simulink model "Model_TranslationEngine64"  (R2022b)
settings: Solver=FixedStepDiscrete  StartTime=0.0  StopTime=5  RelTol=1e-3  EnableMultiTasking=on
InitFcn:
  | % Initialize model
  | ModelSettings=BTConfig.GetModelSettings();
  | 
  | ModelSettings.Validate();
  | 
  | ModelInit;
  | 
  | 
  | % load library data
  | GainLibrary_data;
  | % Load saved values from partition process
  | CapturedConstMask.LoadMapFromFile(bdroot)
StartFcn:
  | % make sure all the simulated RTC requests are found
  | %RTC_SIM_OBJ.ValidateREQs();
undefined symbols (not defined in the file or in its folder): AA, BPLP, Column, NumHFRefBPF, NumHFRefLPF, NumMusicChannels, Row, VolumeMuteConfig
libraries: TuneVar x925, TOP x490, FeaturePath x111, CapturedConstLib x52
(part 28 of 34)

== system Model_TranslationEngine64/ModelPreAmp/DecRate/Medusa5H1/MedusaHoligram/Medusa5H1 Part 3/On/Full-rate Mixer/Full-Rate Mixer with CAE & Fade Ramper/Fade Tuning/Forward Downmix Threshold ==
  TOP : TOP/TOP  TriggerInit=[440 20 585 80]  TopName=ForwardDownmixThreshold  DataTypeOut=single  BankNumber=0  PreOverlay=false  PostOverlay=false  Role=Automatic
      settings: SourceProductName=Bose Talaria
  TranslateTrigger : TuneVar/TranslateTrigger  TriggerInit=[291 -100 329 -45]
      settings: SourceProductName=Bose Talaria
  Trivial Translation : MATLAB Function  TreatAsAtomicUnit=on
  Tune Variable : TuneVar/TuneVar  TuneName=ForwardDownmixThreshold  SpecifyMaxSize=off  VariableDim=1 (Row)  MaxSize=[1 1]  TunabilityNumber=1  MinValue=[0]  MaxValue=[1]  TriggerInit=[-80 25 90 75]  MaskValue=MedusaFRMTune.ForwardDownmixThreshold
      settings: SourceProductName=Bose Talaria
  wires:
  Tune Variable/1 -> Trivial Translation/1(ForwardDownmixThreshold)  "ForwardDownmixThreshold"
  Trivial Translation/1(TOP) -> TOP/1
  TranslateTrigger/1 -> Trivial Translation/Trigger

== system Model_TranslationEngine64/ModelPreAmp/DecRate/Medusa5H1/MedusaHoligram/Medusa5H1 Part 3/On/Full-rate Mixer/Full-Rate Mixer with CAE & Fade Ramper/Fade Tuning/Foward Downmix Max ==
  TOP : TOP/TOP  TriggerInit=[440 20 585 80]  TopName=ForwardDownmixMax  DataTypeOut=single  BankNumber=0  PreOverlay=false  PostOverlay=false  Role=Automatic
      settings: SourceProductName=Bose Talaria
  TranslateTrigger : TuneVar/TranslateTrigger  TriggerInit=[286 -100 324 -45]
      settings: SourceProductName=Bose Talaria
  Trivial Translation : MATLAB Function  TreatAsAtomicUnit=on
  Tune Variable : TuneVar/TuneVar  TuneName=ForwardDownmixMax  SpecifyMaxSize=off  VariableDim=1 (Row)  MaxSize=[1 1]  TunabilityNumber=1  MinValue=[0]  MaxValue=[1]  TriggerInit=[-70 25 100 75]  MaskValue=MedusaFRMTune.ForwardDownmixMax
      settings: SourceProductName=Bose Talaria
  wires:
  Tune Variable/1 -> Trivial Translation/1(ForwardDownmixMax)  "ForwardDownmixMax"
  Trivial Translation/1(TOP) -> TOP/1
  TranslateTrigger/1 -> Trivial Translation/Trigger

== system Model_TranslationEngine64/ModelPreAmp/DecRate/Medusa5H1/MedusaHoligram/Medusa5H1 Part 3/On/Full-rate Mixer/Full-Rate Mixer with CAE & Fade Ramper/SLC Tuning/Detent Level CS ==
  TOP : TOP/TOP  TriggerInit=[440 -15 585 45]  TopName=DetentLevel_CS  DataTypeOut=single  BankNumber=0  PreOverlay=false  PostOverlay=false  Role=Automatic
      settings: SourceProductName=Bose Talaria
  TOP1 : TOP/TOP  TriggerInit=[440 55 585 115]  TopName=DetentLevel_CS_CAE  DataTypeOut=single  BankNumber=0  PreOverlay=false  PostOverlay=false  Role=Automatic
      settings: SourceProductName=Bose Talaria
  TranslateTrigger : TuneVar/TranslateTrigger  TriggerInit=[306 -100 344 -45]
      settings: SourceProductName=Bose Talaria
  Trivial Translation : MATLAB Function  TreatAsAtomicUnit=on
  Tune Variable : TuneVar/TuneVar  TuneName=DetentLevel_CS  SpecifyMaxSize=off  VariableDim=1 (Row)  MaxSize=[1 1]  TunabilityNumber=1  MinValue=[0]  MaxValue=[1]  TriggerInit=[-35 25 135 75]  MaskValue=MedusaFRMTune.detentGain_CS
      settings: SourceProductName=Bose Talaria
  wires:
  Trivial Translation/2(TOP_CAE) -> TOP1/1
  TranslateTrigger/1 -> Trivial Translation/Trigger
  Trivial Translation/1(TOP) -> TOP/1
  Tune Variable/1 -> Trivial Translation/1(detentGain_CS)  "DetentLevel_CS"

== system Model_TranslationEngine64/ModelPreAmp/DecRate/Medusa5H1/MedusaHoligram/Medusa5H1 Part 3/On/Full-rate Mixer/Full-Rate Mixer with CAE & Fade Ramper/SLC Tuning/Detent Level Left ==
  TOP : TOP/TOP  TriggerInit=[440 -15 585 45]  TopName=DetentLevel_Left  DataTypeOut=single  BankNumber=0  PreOverlay=false  PostOverlay=false  Role=Automatic
      settings: SourceProductName=Bose Talaria
  TOP1 : TOP/TOP  TriggerInit=[440 55 585 115]  TopName=DetentLevel_Left_CAE  DataTypeOut=single  BankNumber=0  PreOverlay=false  PostOverlay=false  Role=Automatic
      settings: SourceProductName=Bose Talaria
  TranslateTrigger : TuneVar/TranslateTrigger  TriggerInit=[306 -100 344 -45]
      settings: SourceProductName=Bose Talaria
  Trivial Translation : MATLAB Function  TreatAsAtomicUnit=on
  Tune Variable : TuneVar/TuneVar  TuneName=DetentLevel_Left  SpecifyMaxSize=off  VariableDim=1 (Row)  MaxSize=[1 1]  TunabilityNumber=1  MinValue=[0]  MaxValue=[1]  TriggerInit=[-65 25 105 75]  MaskValue=MedusaFRMTune.detentGain_Left
      settings: SourceProductName=Bose Talaria
  wires:
  Trivial Translation/2(TOP_CAE) -> TOP1/1
  TranslateTrigger/1 -> Trivial Translation/Trigger
  Trivial Translation/1(TOP) -> TOP/1
  Tune Variable/1 -> Trivial Translation/1(detentGain_Left)  "DetentLevel_Left"

== system Model_TranslationEngine64/ModelPreAmp/DecRate/Medusa5H1/MedusaHoligram/Medusa5H1 Part 3/On/Full-rate Mixer/Full-Rate Mixer with CAE & Fade Ramper/SLC Tuning/Detent Level Right ==
  TOP : TOP/TOP  TriggerInit=[440 -15 585 45]  TopName=DetentLevel_Right  DataTypeOut=single  BankNumber=0  PreOverlay=false  PostOverlay=false  Role=Automatic
      settings: SourceProductName=Bose Talaria
  TOP1 : TOP/TOP  TriggerInit=[440 55 585 115]  TopName=DetentLevel_Right_CAE  DataTypeOut=single  BankNumber=0  PreOverlay=false  PostOverlay=false  Role=Automatic
      settings: SourceProductName=Bose Talaria
  TranslateTrigger : TuneVar/TranslateTrigger  TriggerInit=[306 -100 344 -45]
      settings: SourceProductName=Bose Talaria
  Trivial Translation : MATLAB Function  TreatAsAtomicUnit=on
  Tune Variable : TuneVar/TuneVar  TuneName=DetentLevel_Right  SpecifyMaxSize=off  VariableDim=1 (Row)  MaxSize=[1 1]  TunabilityNumber=1  MinValue=[0]  MaxValue=[1]  TriggerInit=[-60 25 110 75]  MaskValue=MedusaFRMTune.detentGain_Right
      settings: SourceProductName=Bose Talaria
  wires:
  Trivial Translation/2(TOP_CAE) -> TOP1/1
  TranslateTrigger/1 -> Trivial Translation/Trigger
  Trivial Translation/1(TOP) -> TOP/1
  Tune Variable/1 -> Trivial Translation/1(detentGain_Right)  "DetentLevel_Right"

== system Model_TranslationEngine64/ModelPreAmp/DecRate/Medusa5H1/MedusaHoligram/Medusa5H1 Part 3/On/Full-rate Mixer/Full-Rate Mixer with CAE & Fade Ramper/SLC Tuning/Interpolation Method ==
  TOP : TOP/TOP  TriggerInit=[440 20 585 80]  TopName=Interpolation_Method  DataTypeOut=single  BankNumber=0  PreOverlay=false  PostOverlay=false  Role=Automatic
      settings: SourceProductName=Bose Talaria
  TranslateTrigger : TuneVar/TranslateTrigger  TriggerInit=[306 -100 344 -45]
      settings: SourceProductName=Bose Talaria
  Trivial Translation : MATLAB Function  TreatAsAtomicUnit=on
  Tune Variable : TuneVar/TuneVar  TuneName=Interpolation_Method  SpecifyMaxSize=off  VariableDim=1 (Row)  MaxSize=[1 1]  TunabilityNumber=2  MinValue=[0]  MaxValue=[1]  TriggerInit=[-40 25 130 75]  MaskValue=MedusaFRMTune.interpolationMethod
      settings: SourceProductName=Bose Talaria
  wires:
  TranslateTrigger/1 -> Trivial Translation/Trigger
  Trivial Translation/1(TOP) -> TOP/1
  Tune Variable/1 -> Trivial Translation/1(interpolationMethod)  "Interpolation_Method"

== system Model_TranslationEngine64/ModelPreAmp/DecRate/Medusa5H1/MedusaHoligram/Medusa5H1 Part 3/On/Full-rate Mixer/Full-Rate Mixer with CAE & Fade Ramper/SLC Tuning/Max Level CS ==
  TOP : TOP/TOP  TriggerInit=[440 -15 585 45]  TopName=MaxLevel_CS  DataTypeOut=single  BankNumber=0  PreOverlay=false  PostOverlay=false  Role=Automatic
      settings: SourceProductName=Bose Talaria
  TOP1 : TOP/TOP  TriggerInit=[440 55 585 115]  TopName=MaxLevel_CS_CAE  DataTypeOut=single  BankNumber=0  PreOverlay=false  PostOverlay=false  Role=Automatic
      settings: SourceProductName=Bose Talaria
  TranslateTrigger : TuneVar/TranslateTrigger  TriggerInit=[306 -100 344 -45]
      settings: SourceProductName=Bose Talaria
  Trivial Translation : MATLAB Function  TreatAsAtomicUnit=on
  Tune Variable : TuneVar/TuneVar  TuneName=MaxLevel_CS  SpecifyMaxSize=off  VariableDim=1 (Row)  MaxSize=[1 1]  TunabilityNumber=1  MinValue=[0]  MaxValue=[1]  TriggerInit=[-45 25 125 75]  MaskValue=MedusaFRMTune.maxGain_CS
      settings: SourceProductName=Bose Talaria
  wires:
  Trivial Translation/2(TOP_CAE) -> TOP1/1
  TranslateTrigger/1 -> Trivial Translation/Trigger
  Trivial Translation/1(TOP) -> TOP/1
  Tune Variable/1 -> Trivial Translation/1(maxGain_CS)  "MaxLevel_CS"

== system Model_TranslationEngine64/ModelPreAmp/DecRate/Medusa5H1/MedusaHoligram/Medusa5H1 Part 3/On/Full-rate Mixer/Full-Rate Mixer with CAE & Fade Ramper/SLC Tuning/Max Level Left ==
  TOP : TOP/TOP  TriggerInit=[440 -15 585 45]  TopName=MaxLevel_Left  DataTypeOut=single  BankNumber=0  PreOverlay=false  PostOverlay=false  Role=Automatic
      settings: SourceProductName=Bose Talaria
  TOP1 : TOP/TOP  TriggerInit=[440 55 585 115]  TopName=MaxLevel_Left_CAE  DataTypeOut=single  BankNumber=0  PreOverlay=false  PostOverlay=false  Role=Automatic
      settings: SourceProductName=Bose Talaria
  TranslateTrigger : TuneVar/TranslateTrigger  TriggerInit=[306 -100 344 -45]
      settings: SourceProductName=Bose Talaria
  Trivial Translation : MATLAB Function  TreatAsAtomicUnit=on
  Tune Variable : TuneVar/TuneVar  TuneName=MaxLevel_Left  SpecifyMaxSize=off  VariableDim=1 (Row)  MaxSize=[1 1]  TunabilityNumber=1  MinValue=[0]  MaxValue=[1]  TriggerInit=[-55 25 115 75]  MaskValue=MedusaFRMTune.maxGain_Left
      settings: SourceProductName=Bose Talaria
  wires:
  Trivial Translation/2(TOP_CAE) -> TOP1/1
  TranslateTrigger/1 -> Trivial Translation/Trigger
  Trivial Translation/1(TOP) -> TOP/1
  Tune Variable/1 -> Trivial Translation/1(maxGain_Left)  "MaxLevel_Left"

== system Model_TranslationEngine64/ModelPreAmp/DecRate/Medusa5H1/MedusaHoligram/Medusa5H1 Part 3/On/Full-rate Mixer/Full-Rate Mixer with CAE & Fade Ramper/SLC Tuning/Max Level Right ==
  TOP : TOP/TOP  TriggerInit=[440 -15 585 45]  TopName=MaxLevel_Right  DataTypeOut=single  BankNumber=0  PreOverlay=false  PostOverlay=false  Role=Automatic
      settings: SourceProductName=Bose Talaria
  TOP1 : TOP/TOP  TriggerInit=[440 55 585 115]  TopName=MaxLevel_Right_CAE  DataTypeOut=single  BankNumber=0  PreOverlay=false  PostOverlay=false  Role=Automatic
      settings: SourceProductName=Bose Talaria
  TranslateTrigger : TuneVar/TranslateTrigger  TriggerInit=[306 -100 344 -45]
      settings: SourceProductName=Bose Talaria
  Trivial Translation : MATLAB Function  TreatAsAtomicUnit=on
  Tune Variable : TuneVar/TuneVar  TuneName=MaxLevel_Right  SpecifyMaxSize=off  VariableDim=1 (Row)  MaxSize=[1 1]  TunabilityNumber=1  MinValue=[0]  MaxValue=[1]  TriggerInit=[-40 25 130 75]  MaskValue=MedusaFRMTune.maxGain_Right
      settings: SourceProductName=Bose Talaria
  wires:
  Trivial Translation/2(TOP_CAE) -> TOP1/1
  TranslateTrigger/1 -> Trivial Translation/Trigger
  Trivial Translation/1(TOP) -> TOP/1
  Tune Variable/1 -> Trivial Translation/1(maxGain_Right)  "MaxLevel_Right"

== system Model_TranslationEngine64/ModelPreAmp/DecRate/Medusa5H1/MedusaHoligram/Medusa5H1 Part 3/On/Full-rate Mixer/Full-Rate Mixer with CAE & Fade Ramper/SLC Tuning/Min Level CS ==
  TOP : TOP/TOP  TriggerInit=[440 -15 585 45]  TopName=MinLevel_CS  DataTypeOut=single  BankNumber=0  PreOverlay=false  PostOverlay=false  Role=Automatic
      settings: SourceProductName=Bose Talaria
  TOP1 : TOP/TOP  TriggerInit=[440 55 585 115]  TopName=MinLevel_CS_CAE  DataTypeOut=single  BankNumber=0  PreOverlay=false  PostOverlay=false  Role=Automatic
      settings: SourceProductName=Bose Talaria
  TranslateTrigger : TuneVar/TranslateTrigger  TriggerInit=[306 -100 344 -45]
      settings: SourceProductName=Bose Talaria
  Trivial Translation : MATLAB Function  TreatAsAtomicUnit=on
  Tune Variable : TuneVar/TuneVar  TuneName=MinLevel_CS  SpecifyMaxSize=off  VariableDim=1 (Row)  MaxSize=[1 1]  TunabilityNumber=1  MinValue=[0]  MaxValue=[1]  TriggerInit=[-45 25 125 75]  MaskValue=MedusaFRMTune.minGain_CS
      settings: SourceProductName=Bose Talaria
  wires:
  Trivial Translation/2(TOP_CAE) -> TOP1/1
  TranslateTrigger/1 -> Trivial Translation/Trigger
  Trivial Translation/1(TOP) -> TOP/1
  Tune Variable/1 -> Trivial Translation/1(minGain_CS)  "MinLevel_CS"

== system Model_TranslationEngine64/ModelPreAmp/DecRate/Medusa5H1/MedusaHoligram/Medusa5H1 Part 3/On/Full-rate Mixer/Full-Rate Mixer with CAE & Fade Ramper/SLC Tuning/Min Level Left ==
  TOP : TOP/TOP  TriggerInit=[380 -90 525 -30]  TopName=MinLevel_Left  DataTypeOut=single  BankNumber=0  PreOverlay=false  PostOverlay=false  Role=Automatic
      settings: SourceProductName=Bose Talaria
  TOP1 : TOP/TOP  TriggerInit=[380 -20 525 40]  TopName=MinLevel_Left_CAE  DataTypeOut=single  BankNumber=0  PreOverlay=false  PostOverlay=false  Role=Automatic
      settings: SourceProductName=Bose Talaria
  TranslateTrigger : TuneVar/TranslateTrigger  TriggerInit=[246 -175 284 -120]
      settings: SourceProductName=Bose Talaria
  Trivial Translation : MATLAB Function  TreatAsAtomicUnit=on
  Tune Variable : TuneVar/TuneVar  TuneName=MinLevel_Left  SpecifyMaxSize=off  VariableDim=1 (Row)  MaxSize=[1 1]  TunabilityNumber=1  MinValue=[0]  MaxValue=[1]  TriggerInit=[-120 -50 50 0]  MaskValue=MedusaFRMTune.minGain_Left
      settings: SourceProductName=Bose Talaria
  wires:
  Trivial Translation/2(TOP_CAE) -> TOP1/1
  TranslateTrigger/1 -> Trivial Translation/Trigger
  Trivial Translation/1(TOP) -> TOP/1
  Tune Variable/1 -> Trivial Translation/1(minGain_Left)  "MinLevel_Left"

== system Model_TranslationEngine64/ModelPreAmp/DecRate/Medusa5H1/MedusaHoligram/Medusa5H1 Part 3/On/Full-rate Mixer/Full-Rate Mixer with CAE & Fade Ramper/SLC Tuning/Min Level Right ==
  TOP : TOP/TOP  TriggerInit=[440 -15 585 45]  TopName=MinLevel_Right  DataTypeOut=single  BankNumber=0  PreOverlay=false  PostOverlay=false  Role=Automatic
      settings: SourceProductName=Bose Talaria
  TOP1 : TOP/TOP  TriggerInit=[440 55 585 115]  TopName=MinLevel_Right_CAE  DataTypeOut=single  BankNumber=0  PreOverlay=false  PostOverlay=false  Role=Automatic
      settings: SourceProductName=Bose Talaria
  TranslateTrigger : TuneVar/TranslateTrigger  TriggerInit=[306 -100 344 -45]
      settings: SourceProductName=Bose Talaria
  Trivial Translation : MATLAB Function  TreatAsAtomicUnit=on
  Tune Variable : TuneVar/TuneVar  TuneName=MinLevel_Right  SpecifyMaxSize=off  VariableDim=1 (Row)  MaxSize=[1 1]  TunabilityNumber=1  MinValue=[0]  MaxValue=[1]  TriggerInit=[-40 25 130 75]  MaskValue=MedusaFRMTune.minGain_Right
      settings: SourceProductName=Bose Talaria
  wires:
  Trivial Translation/2(TOP_CAE) -> TOP1/1
  TranslateTrigger/1 -> Trivial Translation/Trigger
  Trivial Translation/1(TOP) -> TOP/1
  Tune Variable/1 -> Trivial Translation/1(minGain_Right)  "MinLevel_Right"

== system Model_TranslationEngine64/ModelPreAmp/DecRate/Medusa5H1/MedusaHoligram/Medusa5H1 Part 3/On/Premix/Premix with Mono-Surround & CAE with Fade Ramper/CS Processing/MS Tune ==
  TOP : TOP/TOP  TriggerInit=[260 -150 405 -90]  TopName=Phi  DataTypeOut=single  BankNumber=0  PreOverlay=false  PostOverlay=false  Role=Automatic
      settings: SourceProductName=Bose Talaria
  TOP1 : TOP/TOP  TriggerInit=[260 -70 405 -10]  TopName=CosPhi  DataTypeOut=single  BankNumber=0  PreOverlay=false  PostOverlay=false  Role=Automatic
      settings: SourceProductName=Bose Talaria
  TOP2 : TOP/TOP  TriggerInit=[260 10 405 70]  TopName=SinPhi  DataTypeOut=single  BankNumber=0  PreOverlay=false  PostOverlay=false  Role=Automatic
      settings: SourceProductName=Bose Talaria
  TranslateTrigger : TuneVar/TranslateTrigger  TriggerInit=[66 -245 104 -190]
      settings: SourceProductName=Bose Talaria
  Tune Variable : TuneVar/TuneVar  TuneName=PhaseAngle  SpecifyMaxSize=off  VariableDim=1 (Row)  MaxSize=[1 1]  TunabilityNumber=1  MinValue=[]  MaxValue=[]  TriggerInit=[-270 -65 -100 -15]  MaskValue=MSConfig.DefaultPhaseAngle
      settings: SourceProductName=Bose Talaria
  translation : MATLAB Function  TreatAsAtomicUnit=on
  wires:
  translation/3(sin_phi) -> TOP2/1
  translation/2(cos_phi) -> TOP1/1
  Tune Variable/1 -> translation/1(PhaseAngle)  "PhaseAngle"
  TranslateTrigger/1 -> translation/Trigger
  translation/1(phi) -> TOP/1

== system Model_TranslationEngine64/ModelPreAmp/DecRate/Medusa5H1/MedusaHoligram/Medusa5H1 Part 3/On/Premix/Premix with Mono-Surround & CAE with Fade Ramper/Fade Tuning/Backward Downmix Max ==
  TOP : TOP/TOP  TriggerInit=[440 20 585 80]  TopName=BackwardDownmixMax  DataTypeOut=single  BankNumber=0  PreOverlay=false  PostOverlay=false  Role=Automatic
      settings: SourceProductName=Bose Talaria
  TranslateTrigger : TuneVar/TranslateTrigger  TriggerInit=[286 -100 324 -45]
      settings: SourceProductName=Bose Talaria
  Trivial Translation : MATLAB Function  TreatAsAtomicUnit=on
  Tune Variable : TuneVar/TuneVar  TuneName=BackwardDownmixMax  SpecifyMaxSize=off  VariableDim=1 (Row)  MaxSize=[1 1]  TunabilityNumber=1  MinValue=[0]  MaxValue=[1]  TriggerInit=[-65 25 105 75]  MaskValue=MedusaPremixTune.BackwardDownmixMax
      settings: SourceProductName=Bose Talaria
  wires:
  TranslateTrigger/1 -> Trivial Translation/Trigger
  Trivial Translation/1(TOP) -> TOP/1
  Tune Variable/1 -> Trivial Translation/1(BackwardDownmixMax)  "BackwardDownmixMax"

== system Model_TranslationEngine64/ModelPreAmp/DecRate/Medusa5H1/MedusaHoligram/Medusa5H1 Part 3/On/Premix/Premix with Mono-Surround & CAE with Fade Ramper/Fade Tuning/Backward Downmix Threshold ==
  TOP : TOP/TOP  TriggerInit=[440 20 585 80]  TopName=BackwardDownmixThreshold  DataTypeOut=single  BankNumber=0  PreOverlay=false  PostOverlay=false  Role=Automatic
      settings: SourceProductName=Bose Talaria
  TranslateTrigger : TuneVar/TranslateTrigger  TriggerInit=[306 -100 344 -45]
      settings: SourceProductName=Bose Talaria
  Trivial Translation : MATLAB Function  TreatAsAtomicUnit=on
  Tune Variable : TuneVar/TuneVar  TuneName=BackwardDownmixThreshold  SpecifyMaxSize=off  VariableDim=1 (Row)  MaxSize=[1 1]  TunabilityNumber=1  MinValue=[0]  MaxValue=[1]  TriggerInit=[-75 25 95 75]  MaskValue=MedusaPremixTune.BackwardDownmixThreshold
      settings: SourceProductName=Bose Talaria
  wires:
  TranslateTrigger/1 -> Trivial Translation/Trigger
  Trivial Translation/1(TOP) -> TOP/1
  Tune Variable/1 -> Trivial Translation/1(BackwardDownmixThreshold)  "BackwardDownmixThreshold"

== system Model_TranslationEngine64/ModelPreAmp/DecRate/Medusa5H1/MedusaHoligram/Medusa5H1 Part 3/On/Premix/Premix with Mono-Surround & CAE with Fade Ramper/Fade Tuning/Downmix Weights CS ==
  TOP : TOP/TOP  TriggerInit=[440 -15 600 45]  TopName=DownmixWeights_CS  DataTypeOut=single  BankNumber=0  PreOverlay=false  PostOverlay=false  Role=Automatic
      settings: SourceProductName=Bose Talaria
  TOP1 : TOP/TOP  TriggerInit=[440 55 600 115]  TopName=DownmixWeights_CS_CAE  DataTypeOut=single  BankNumber=0  PreOverlay=false  PostOverlay=false  Role=Automatic
      settings: SourceProductName=Bose Talaria
  TranslateTrigger : TuneVar/TranslateTrigger  TriggerInit=[256 -100 294 -45]
      settings: SourceProductName=Bose Talaria
  Trivial Translation : MATLAB Function  TreatAsAtomicUnit=on
  Tune Variable : TuneVar/TuneVar  TuneName=DownmixWeights_CS  SpecifyMaxSize=off  VariableDim=1 (Row)  MaxSize=[1 1]  TunabilityNumber=1  MinValue=[0]  MaxValue=[1]  TriggerInit=[-85 25 85 75]  MaskValue=MedusaPremixTune.downmix_wts_CS
      settings: SourceProductName=Bose Talaria
  wires:
  Trivial Translation/2(TOP_CAE) -> TOP1/1
  TranslateTrigger/1 -> Trivial Translation/Trigger
  Trivial Translation/1(TOP) -> TOP/1
  Tune Variable/1 -> Trivial Translation/1(downmix_wts_CS)  "DownmixWeights_CS"

== system Model_TranslationEngine64/ModelPreAmp/DecRate/Medusa5H1/MedusaHoligram/Medusa5H1 Part 3/On/Premix/Premix with Mono-Surround & CAE with Fade Ramper/Fade Tuning/Downmix Weights Left ==
  TOP : TOP/TOP  TriggerInit=[440 -15 605 45]  TopName=DownmixWeights_Left  DataTypeOut=single  BankNumber=0  PreOverlay=false  PostOverlay=false  Role=Automatic
      settings: SourceProductName=Bose Talaria
  TOP1 : TOP/TOP  TriggerInit=[440 55 605 115]  TopName=DownmixWeights_Left_CAE  DataTypeOut=single  BankNumber=0  PreOverlay=false  PostOverlay=false  Role=Automatic
      settings: SourceProductName=Bose Talaria
  TranslateTrigger : TuneVar/TranslateTrigger  TriggerInit=[266 -100 304 -45]
      settings: SourceProductName=Bose Talaria
  Trivial Translation : MATLAB Function  TreatAsAtomicUnit=on
  Tune Variable : TuneVar/TuneVar  TuneName=DownmixWeights_Left  SpecifyMaxSize=off  VariableDim=1 (Row)  MaxSize=[1 1]  TunabilityNumber=1  MinValue=[0]  MaxValue=[1]  TriggerInit=[-80 25 90 75]  MaskValue=MedusaPremixTune.downmix_wts_Left
      settings: SourceProductName=Bose Talaria
  wires:
  Trivial Translation/2(TOP_CAE) -> TOP1/1
  TranslateTrigger/1 -> Trivial Translation/Trigger
  Trivial Translation/1(TOP) -> TOP/1
  Tune Variable/1 -> Trivial Translation/1(downmix_wts_Left)  "DownmixWeights_Left"

== system Model_TranslationEngine64/ModelPreAmp/DecRate/Medusa5H1/MedusaHoligram/Medusa5H1 Part 3/On/Premix/Premix with Mono-Surround & CAE with Fade Ramper/Fade Tuning/Downmix Weights Right ==
  TOP : TOP/TOP  TriggerInit=[475 -15 645 45]  TopName=DownmixWeights_Right  DataTypeOut=single  BankNumber=0  PreOverlay=false  PostOverlay=false  Role=Automatic
      settings: SourceProductName=Bose Talaria
  TOP1 : TOP/TOP  TriggerInit=[475 55 645 115]  TopName=DownmixWeights_Right_CAE  DataTypeOut=single  BankNumber=0  PreOverlay=false  PostOverlay=false  Role=Automatic
      settings: SourceProductName=Bose Talaria
  TranslateTrigger : TuneVar/TranslateTrigger  TriggerInit=[306 -100 344 -45]
      settings: SourceProductName=Bose Talaria
  Trivial Translation : MATLAB Function  TreatAsAtomicUnit=on
  Tune Variable : TuneVar/TuneVar  TuneName=DownmixWeights_Right  SpecifyMaxSize=off  VariableDim=1 (Row)  MaxSize=[1 1]  TunabilityNumber=1  MinValue=[0]  MaxValue=[1]  TriggerInit=[-40 25 130 75]  MaskValue=MedusaPremixTune.downmix_wts_Right
      settings: SourceProductName=Bose Talaria
  wires:
  Trivial Translation/2(TOP_CAE) -> TOP1/1
  TranslateTrigger/1 -> Trivial Translation/Trigger
  Trivial Translation/1(TOP) -> TOP/1
  Tune Variable/1 -> Trivial Translation/1(downmix_wts_Right)  "DownmixWeights_Right"

== system Model_TranslationEngine64/ModelPreAmp/DecRate/Medusa5H1/MedusaHoligram/Medusa5H1 Part 3/On/Premix/Premix with Mono-Surround & CAE with Fade Ramper/Fade Tuning/Forward Downmix Threshold ==
  TOP : TOP/TOP  TriggerInit=[440 20 585 80]  TopName=ForwardDownmixThreshold  DataTypeOut=single  BankNumber=0  PreOverlay=false  PostOverlay=false  Role=Automatic
      settings: SourceProductName=Bose Talaria
  TranslateTrigger : TuneVar/TranslateTrigger  TriggerInit=[291 -100 329 -45]
      settings: SourceProductName=Bose Talaria
  Trivial Translation : MATLAB Function  TreatAsAtomicUnit=on
  Tune Variable : TuneVar/TuneVar  TuneName=ForwardDownmixThreshold  SpecifyMaxSize=off  VariableDim=1 (Row)  MaxSize=[1 1]  TunabilityNumber=1  MinValue=[0]  MaxValue=[1]  TriggerInit=[-80 25 90 75]  MaskValue=MedusaPremixTune.ForwardDownmixThreshold
      settings: SourceProductName=Bose Talaria
  wires:
  TranslateTrigger/1 -> Trivial Translation/Trigger
  Trivial Translation/1(TOP) -> TOP/1
  Tune Variable/1 -> Trivial Translation/1(ForwardDownmixThreshold)  "ForwardDownmixThreshold"

== system Model_TranslationEngine64/ModelPreAmp/DecRate/Medusa5H1/MedusaHoligram/Medusa5H1 Part 3/On/Premix/Premix with Mono-Surround & CAE with Fade Ramper/Fade Tuning/Foward Downmix Max ==
  TOP : TOP/TOP  TriggerInit=[440 20 585 80]  TopName=ForwardDownmixMax  DataTypeOut=single  BankNumber=0  PreOverlay=false  PostOverlay=false  Role=Automatic
      settings: SourceProductName=Bose Talaria
  TranslateTrigger : TuneVar/TranslateTrigger  TriggerInit=[286 -100 324 -45]
      settings: SourceProductName=Bose Talaria
  Trivial Translation : MATLAB Function  TreatAsAtomicUnit=on
  Tune Variable : TuneVar/TuneVar  TuneName=ForwardDownmixMax  SpecifyMaxSize=off  VariableDim=1 (Row)  MaxSize=[1 1]  TunabilityNumber=1  MinValue=[0]  MaxValue=[1]  TriggerInit=[-70 25 100 75]  MaskValue=MedusaPremixTune.ForwardDownmixMax
      settings: SourceProductName=Bose Talaria
  wires:
  TranslateTrigger/1 -> Trivial Translation/Trigger
  Trivial Translation/1(TOP) -> TOP/1
  Tune Variable/1 -> Trivial Translation/1(ForwardDownmixMax)  "ForwardDownmixMax"

== system Model_TranslationEngine64/ModelPreAmp/DecRate/Medusa5H1/MedusaHoligram/Medusa5H1 Part 3/On/Premix/Premix with Mono-Surround & CAE with Fade Ramper/SLC Tuning/Detent Level CS ==
  TOP : TOP/TOP  TriggerInit=[440 -15 585 45]  TopName=DetentLevel_CS  DataTypeOut=single  BankNumber=0  PreOverlay=false  PostOverlay=false  Role=Automatic
      settings: SourceProductName=Bose Talaria
  TOP1 : TOP/TOP  TriggerInit=[440 55 585 115]  TopName=DetentLevel_CS_CAE  DataTypeOut=single  BankNumber=0  PreOverlay=false  PostOverlay=false  Role=Automatic
      settings: SourceProductName=Bose Talaria
  TranslateTrigger : TuneVar/TranslateTrigger  TriggerInit=[306 -100 344 -45]
      settings: SourceProductName=Bose Talaria
  Trivial Translation : MATLAB Function  TreatAsAtomicUnit=on
  Tune Variable : TuneVar/TuneVar  TuneName=DetentLevel_CS  SpecifyMaxSize=off  VariableDim=1 (Row)  MaxSize=[1 1]  TunabilityNumber=1  MinValue=[0]  MaxValue=[1]  TriggerInit=[-35 25 135 75]  MaskValue=MedusaPremixTune.detentGain_CS
      settings: SourceProductName=Bose Talaria
  wires:
  Tune Variable/1 -> Trivial Translation/1(detentGain_CS)  "DetentLevel_CS"
  Trivial Translation/1(TOP) -> TOP/1
  TranslateTrigger/1 -> Trivial Translation/Trigger
  Trivial Translation/2(TOP_CAE) -> TOP1/1

== system Model_TranslationEngine64/ModelPreAmp/DecRate/Medusa5H1/MedusaHoligram/Medusa5H1 Part 3/On/Premix/Premix with Mono-Surround & CAE with Fade Ramper/SLC Tuning/Detent Level Left ==
  TOP : TOP/TOP  TriggerInit=[440 -15 585 45]  TopName=DetentLevel_Left  DataTypeOut=single  BankNumber=0  PreOverlay=false  PostOverlay=false  Role=Automatic
      settings: SourceProductName=Bose Talaria
  TOP1 : TOP/TOP  TriggerInit=[440 55 585 115]  TopName=DetentLevel_Left_CAE  DataTypeOut=single  BankNumber=0  PreOverlay=false  PostOverlay=false  Role=Automatic
      settings: SourceProductName=Bose Talaria
  TranslateTrigger : TuneVar/TranslateTrigger  TriggerInit=[306 -100 344 -45]
      settings: SourceProductName=Bose Talaria
  Trivial Translation : MATLAB Function  TreatAsAtomicUnit=on
  Tune Variable : TuneVar/TuneVar  TuneName=DetentLevel_Left  SpecifyMaxSize=off  VariableDim=1 (Row)  MaxSize=[1 1]  TunabilityNumber=1  MinValue=[0]  MaxValue=[1]  TriggerInit=[-65 25 105 75]  MaskValue=MedusaPremixTune.detentGain_Left
      settings: SourceProductName=Bose Talaria
  wires:
  Tune Variable/1 -> Trivial Translation/1(detentGain_Left)  "DetentLevel_Left"
  Trivial Translation/1(TOP) -> TOP/1
  TranslateTrigger/1 -> Trivial Translation/Trigger
  Trivial Translation/2(TOP_CAE) -> TOP1/1

== system Model_TranslationEngine64/ModelPreAmp/DecRate/Medusa5H1/MedusaHoligram/Medusa5H1 Part 3/On/Premix/Premix with Mono-Surround & CAE with Fade Ramper/SLC Tuning/Detent Level Right ==
  TOP : TOP/TOP  TriggerInit=[440 -15 585 45]  TopName=DetentLevel_Right  DataTypeOut=single  BankNumber=0  PreOverlay=false  PostOverlay=false  Role=Automatic
      settings: SourceProductName=Bose Talaria
  TOP1 : TOP/TOP  TriggerInit=[440 55 585 115]  TopName=DetentLevel_Right_CAE  DataTypeOut=single  BankNumber=0  PreOverlay=false  PostOverlay=false  Role=Automatic
      settings: SourceProductName=Bose Talaria
  TranslateTrigger : TuneVar/TranslateTrigger  TriggerInit=[306 -100 344 -45]
      settings: SourceProductName=Bose Talaria
  Trivial Translation : MATLAB Function  TreatAsAtomicUnit=on
  Tune Variable : TuneVar/TuneVar  TuneName=DetentLevel_Right  SpecifyMaxSize=off  VariableDim=1 (Row)  MaxSize=[1 1]  TunabilityNumber=1  MinValue=[0]  MaxValue=[1]  TriggerInit=[-60 25 110 75]  MaskValue=MedusaPremixTune.detentGain_Right
      settings: SourceProductName=Bose Talaria
  wires:
  Tune Variable/1 -> Trivial Translation/1(detentGain_Right)  "DetentLevel_Right"
  Trivial Translation/1(TOP) -> TOP/1
  TranslateTrigger/1 -> Trivial Translation/Trigger
  Trivial Translation/2(TOP_CAE) -> TOP1/1

== system Model_TranslationEngine64/ModelPreAmp/DecRate/Medusa5H1/MedusaHoligram/Medusa5H1 Part 3/On/Premix/Premix with Mono-Surround & CAE with Fade Ramper/SLC Tuning/Interpolation Method ==
  TOP : TOP/TOP  TriggerInit=[440 20 585 80]  TopName=Interpolation_Method  DataTypeOut=single  BankNumber=0  PreOverlay=false  PostOverlay=false  Role=Automatic
      settings: SourceProductName=Bose Talaria
  TranslateTrigger : TuneVar/TranslateTrigger  TriggerInit=[306 -100 344 -45]
      settings: SourceProductName=Bose Talaria
  Trivial Translation : MATLAB Function  TreatAsAtomicUnit=on
  Tune Variable : TuneVar/TuneVar  TuneName=Interpolation_Method  SpecifyMaxSize=off  VariableDim=1 (Row)  MaxSize=[1 1]  TunabilityNumber=2  MinValue=[0]  MaxValue=[1]  TriggerInit=[-40 25 130 75]  MaskValue=MedusaPremixTune.interpolationMethod
      settings: SourceProductName=Bose Talaria
  wires:
  Tune Variable/1 -> Trivial Translation/1(interpolationMethod)  "Interpolation_Method"
  Trivial Translation/1(TOP) -> TOP/1
  TranslateTrigger/1 -> Trivial Translation/Trigger

== system Model_TranslationEngine64/ModelPreAmp/DecRate/Medusa5H1/MedusaHoligram/Medusa5H1 Part 3/On/Premix/Premix with Mono-Surround & CAE with Fade Ramper/SLC Tuning/Max Level CS ==
  TOP : TOP/TOP  TriggerInit=[440 -15 585 45]  TopName=MaxLevel_CS  DataTypeOut=single  BankNumber=0  PreOverlay=false  PostOverlay=false  Role=Automatic
      settings: SourceProductName=Bose Talaria
  TOP1 : TOP/TOP  TriggerInit=[440 55 585 115]  TopName=MaxLevel_CS_CAE  DataTypeOut=single  BankNumber=0  PreOverlay=false  PostOverlay=false  Role=Automatic
      settings: SourceProductName=Bose Talaria
  TranslateTrigger : TuneVar/TranslateTrigger  TriggerInit=[306 -100 344 -45]
      settings: SourceProductName=Bose Talaria
  Trivial Translation : MATLAB Function  TreatAsAtomicUnit=on
  Tune Variable : TuneVar/TuneVar  TuneName=MaxLevel_CS  SpecifyMaxSize=off  VariableDim=1 (Row)  MaxSize=[1 1]  TunabilityNumber=1  MinValue=[0]  MaxValue=[1]  TriggerInit=[-45 25 125 75]  MaskValue=MedusaPremixTune.maxGain_CS
      settings: SourceProductName=Bose Talaria
  wires:
  Tune Variable/1 -> Trivial Translation/1(maxGain_CS)  "MaxLevel_CS"
  Trivial Translation/1(TOP) -> TOP/1
  TranslateTrigger/1 -> Trivial Translation/Trigger
  Trivial Translation/2(TOP_CAE) -> TOP1/1

== system Model_TranslationEngine64/ModelPreAmp/DecRate/Medusa5H1/MedusaHoligram/Medusa5H1 Part 3/On/Premix/Premix with Mono-Surround & CAE with Fade Ramper/SLC Tuning/Max Level Left ==
  TOP : TOP/TOP  TriggerInit=[440 -15 585 45]  TopName=MaxLevel_Left  DataTypeOut=single  BankNumber=0  PreOverlay=false  PostOverlay=false  Role=Automatic
      settings: SourceProductName=Bose Talaria
  TOP1 : TOP/TOP  TriggerInit=[440 55 585 115]  TopName=MaxLevel_Left_CAE  DataTypeOut=single  BankNumber=0  PreOverlay=false  PostOverlay=false  Role=Automatic
      settings: SourceProductName=Bose Talaria
  TranslateTrigger : TuneVar/TranslateTrigger  TriggerInit=[306 -100 344 -45]
      settings: SourceProductName=Bose Talaria
  Trivial Translation : MATLAB Function  TreatAsAtomicUnit=on
  Tune Variable : TuneVar/TuneVar  TuneName=MaxLevel_Left  SpecifyMaxSize=off  VariableDim=1 (Row)  MaxSize=[1 1]  TunabilityNumber=1  MinValue=[0]  MaxValue=[1]  TriggerInit=[-55 25 115 75]  MaskValue=MedusaPremixTune.maxGain_Left
      settings: SourceProductName=Bose Talaria
  wires:
  Tune Variable/1 -> Trivial Translation/1(maxGain_Left)  "MaxLevel_Left"
  Trivial Translation/1(TOP) -> TOP/1
  TranslateTrigger/1 -> Trivial Translation/Trigger
  Trivial Translation/2(TOP_CAE) -> TOP1/1

== system Model_TranslationEngine64/ModelPreAmp/DecRate/Medusa5H1/MedusaHoligram/Medusa5H1 Part 3/On/Premix/Premix with Mono-Surround & CAE with Fade Ramper/SLC Tuning/Max Level Right ==
  TOP : TOP/TOP  TriggerInit=[440 -15 585 45]  TopName=MaxLevel_Right  DataTypeOut=single  BankNumber=0  PreOverlay=false  PostOverlay=false  Role=Automatic
      settings: SourceProductName=Bose Talaria
  TOP1 : TOP/TOP  TriggerInit=[440 55 585 115]  TopName=MaxLevel_Right_CAE  DataTypeOut=single  BankNumber=0  PreOverlay=false  PostOverlay=false  Role=Automatic
      settings: SourceProductName=Bose Talaria
  TranslateTrigger : TuneVar/TranslateTrigger  TriggerInit=[306 -100 344 -45]
      settings: SourceProductName=Bose Talaria
  Trivial Translation : MATLAB Function  TreatAsAtomicUnit=on
  Tune Variable : TuneVar/TuneVar  TuneName=MaxLevel_Right  SpecifyMaxSize=off  VariableDim=1 (Row)  MaxSize=[1 1]  TunabilityNumber=1  MinValue=[0]  MaxValue=[1]  TriggerInit=[-40 25 130 75]  MaskValue=MedusaPremixTune.maxGain_Right
      settings: SourceProductName=Bose Talaria
  wires:
  Tune Variable/1 -> Trivial Translation/1(maxGain_Right)  "MaxLevel_Right"
  Trivial Translation/1(TOP) -> TOP/1
  TranslateTrigger/1 -> Trivial Translation/Trigger
  Trivial Translation/2(TOP_CAE) -> TOP1/1

== system Model_TranslationEngine64/ModelPreAmp/DecRate/Medusa5H1/MedusaHoligram/Medusa5H1 Part 3/On/Premix/Premix with Mono-Surround & CAE with Fade Ramper/SLC Tuning/Min Level CS ==
  TOP : TOP/TOP  TriggerInit=[440 -15 585 45]  TopName=MinLevel_CS  DataTypeOut=single  BankNumber=0  PreOverlay=false  PostOverlay=false  Role=Automatic
      settings: SourceProductName=Bose Talaria
  TOP1 : TOP/TOP  TriggerInit=[440 55 585 115]  TopName=MinLevel_CS_CAE  DataTypeOut=single  BankNumber=0  PreOverlay=false  PostOverlay=false  Role=Automatic
      settings: SourceProductName=Bose Talaria
  TranslateTrigger : TuneVar/TranslateTrigger  TriggerInit=[306 -100 344 -45]
      settings: SourceProductName=Bose Talaria
  Trivial Translation : MATLAB Function  TreatAsAtomicUnit=on
  Tune Variable : TuneVar/TuneVar  TuneName=MinLevel_CS  SpecifyMaxSize=off  VariableDim=1 (Row)  MaxSize=[1 1]  TunabilityNumber=1  MinValue=[0]  MaxValue=[1]  TriggerInit=[-45 25 125 75]  MaskValue=MedusaPremixTune.minGain_CS
      settings: SourceProductName=Bose Talaria
  wires:
  Tune Variable/1 -> Trivial Translation/1(minGain_CS)  "MinLevel_CS"
  Trivial Translation/1(TOP) -> TOP/1
  TranslateTrigger/1 -> Trivial Translation/Trigger
  Trivial Translation/2(TOP_CAE) -> TOP1/1

== system Model_TranslationEngine64/ModelPreAmp/DecRate/Medusa5H1/MedusaHoligram/Medusa5H1 Part 3/On/Premix/Premix with Mono-Surround & CAE with Fade Ramper/SLC Tuning/Min Level Left ==
  TOP : TOP/TOP  TriggerInit=[380 -20 525 40]  TopName=MinLevel_Left  DataTypeOut=single  BankNumber=0  PreOverlay=false  PostOverlay=false  Role=Automatic
      settings: SourceProductName=Bose Talaria
  TOP1 : TOP/TOP  TriggerInit=[380 50 525 110]  TopName=MinLevel_Left_CAE  DataTypeOut=single  BankNumber=0  PreOverlay=false  PostOverlay=false  Role=Automatic
      settings: SourceProductName=Bose Talaria
  TranslateTrigger : TuneVar/TranslateTrigger  TriggerInit=[246 -105 284 -50]
      settings: SourceProductName=Bose Talaria
  Trivial Translation : MATLAB Function  TreatAsAtomicUnit=on
  Tune Variable : TuneVar/TuneVar  TuneName=MinLevel_Left  SpecifyMaxSize=off  VariableDim=1 (Row)  MaxSize=[1 1]  TunabilityNumber=1  MinValue=[0]  MaxValue=[1]  TriggerInit=[-120 20 50 70]  MaskValue=MedusaPremixTune.minGain_Left
      settings: SourceProductName=Bose Talaria
  wires:
  Tune Variable/1 -> Trivial Translation/1(minGain_Left)  "MinLevel_Left"
  Trivial Translation/1(TOP) -> TOP/1
  TranslateTrigger/1 -> Trivial Translation/Trigger
  Trivial Translation/2(TOP_CAE) -> TOP1/1

== system Model_TranslationEngine64/ModelPreAmp/DecRate/Medusa5H1/MedusaHoligram/Medusa5H1 Part 3/On/Premix/Premix with Mono-Surround & CAE with Fade Ramper/SLC Tuning/Min Level Right ==
  TOP : TOP/TOP  TriggerInit=[440 -15 585 45]  TopName=MinLevel_Right  DataTypeOut=single  BankNumber=0  PreOverlay=false  PostOverlay=false  Role=Automatic
      settings: SourceProductName=Bose Talaria
  TOP1 : TOP/TOP  TriggerInit=[440 55 585 115]  TopName=MinLevel_Right_CAE  DataTypeOut=single  BankNumber=0  PreOverlay=false  PostOverlay=false  Role=Automatic
      settings: SourceProductName=Bose Talaria
  TranslateTrigger : TuneVar/TranslateTrigger  TriggerInit=[306 -100 344 -45]
      settings: SourceProductName=Bose Talaria
  Trivial Translation : MATLAB Function  TreatAsAtomicUnit=on
  Tune Variable : TuneVar/TuneVar  TuneName=MinLevel_Right  SpecifyMaxSize=off  VariableDim=1 (Row)  MaxSize=[1 1]  TunabilityNumber=1  MinValue=[0]  MaxValue=[1]  TriggerInit=[-40 25 130 75]  MaskValue=MedusaPremixTune.minGain_Right
      settings: SourceProductName=Bose Talaria
  wires:
  Tune Variable/1 -> Trivial Translation/1(minGain_Right)  "MinLevel_Right"
  Trivial Translation/1(TOP) -> TOP/1
  TranslateTrigger/1 -> Trivial Translation/Trigger
  Trivial Translation/2(TOP_CAE) -> TOP1/1

== system Model_TranslationEngine64/ModelPreAmp/DecRate/Medusa5H1/MedusaHoligram/Medusa5H1 Part 3/On/VLS Gains Computation/VLS Gains Drv/Fade Tuning/Backward Downmix Max ==
  TOP : TOP/TOP  TriggerInit=[440 20 585 80]  TopName=BackwardDownmixMax  DataTypeOut=single  BankNumber=0  PreOverlay=false  PostOverlay=false  Role=Automatic
      settings: SourceProductName=Bose Talaria
  TranslateTrigger : TuneVar/TranslateTrigger  TriggerInit=[286 -100 324 -45]
      settings: SourceProductName=Bose Talaria
  Trivial Translation : MATLAB Function  TreatAsAtomicUnit=on
  Tune Variable : TuneVar/TuneVar  TuneName=BackwardDownmixMax  SpecifyMaxSize=off  VariableDim=1 (Row)  MaxSize=[1 1]  TunabilityNumber=1  MinValue=[0]  MaxValue=[1]  TriggerInit=[-65 25 105 75]  MaskValue=tuneStruct.BackwardDownmixMax
      settings: SourceProductName=Bose Talaria
  wires:
  Tune Variable/1 -> Trivial Translation/1(BackwardDownmixMax)  "BackwardDownmixMax"
  Trivial Translation/1(TOP) -> TOP/1
  TranslateTrigger/1 -> Trivial Translation/Trigger

== system Model_TranslationEngine64/ModelPreAmp/DecRate/Medusa5H1/MedusaHoligram/Medusa5H1 Part 3/On/VLS Gains Computation/VLS Gains Drv/Fade Tuning/Backward Downmix Threshold ==
  TOP : TOP/TOP  TriggerInit=[440 20 585 80]  TopName=BackwardDownmixThreshold  DataTypeOut=single  BankNumber=0  PreOverlay=false  PostOverlay=false  Role=Automatic
      settings: SourceProductName=Bose Talaria
  TranslateTrigger : TuneVar/TranslateTrigger  TriggerInit=[306 -100 344 -45]
      settings: SourceProductName=Bose Talaria
  Trivial Translation : MATLAB Function  TreatAsAtomicUnit=on
  Tune Variable : TuneVar/TuneVar  TuneName=BackwardDownmixThreshold  SpecifyMaxSize=off  VariableDim=1 (Row)  MaxSize=[1 1]  TunabilityNumber=1  MinValue=[0]  MaxValue=[1]  TriggerInit=[-75 25 95 75]  MaskValue=tuneStruct.BackwardDownmixThreshold
      settings: SourceProductName=Bose Talaria
  wires:
  Tune Variable/1 -> Trivial Translation/1(BackwardDownmixThreshold)  "BackwardDownmixThreshold"
  Trivial Translation/1(TOP) -> TOP/1
  TranslateTrigger/1 -> Trivial Translation/Trigger

== system Model_TranslationEngine64/ModelPreAmp/DecRate/Medusa5H1/MedusaHoligram/Medusa5H1 Part 3/On/VLS Gains Computation/VLS Gains Drv/Fade Tuning/Downmix Weights ==
  TOP : TOP/TOP  TriggerInit=[385 17 610 83]  TopName=DownmixWeights  DataTypeOut=single  BankNumber=0  PreOverlay=false  PostOverlay=false  Role=Automatic
      settings: SourceProductName=Bose Talaria
  TranslateTrigger : TuneVar/TranslateTrigger  TriggerInit=[266 -100 304 -45]
      settings: SourceProductName=Bose Talaria
  Trivial Translation : MATLAB Function  TreatAsAtomicUnit=on
  Tune Variable : TuneVar/TuneVar  TuneName=DownmixWeights  SpecifyMaxSize=off  VariableDim=1 (Row)  MaxSize=[1 1]  TunabilityNumber=1  MinValue=[0]  MaxValue=[1]  TriggerInit=[-80 25 150 75]  MaskValue=tuneStruct.downmix_wts
      settings: SourceProductName=Bose Talaria
  wires:
  Tune Variable/1 -> Trivial Translation/1(downmix_wts)  "DownmixWeights"
  Trivial Translation/1(TOP) -> TOP/1
  TranslateTrigger/1 -> Trivial Translation/Trigger

== system Model_TranslationEngine64/ModelPreAmp/DecRate/Medusa5H1/MedusaHoligram/Medusa5H1 Part 3/On/VLS Gains Computation/VLS Gains Drv/Fade Tuning/Forward Downmix Threshold ==
  TOP : TOP/TOP  TriggerInit=[440 20 585 80]  TopName=ForwardDownmixThreshold  DataTypeOut=single  BankNumber=0  PreOverlay=false  PostOverlay=false  Role=Automatic
      settings: SourceProductName=Bose Talaria
  TranslateTrigger : TuneVar/TranslateTrigger  TriggerInit=[291 -100 329 -45]
      settings: SourceProductName=Bose Talaria
  Trivial Translation : MATLAB Function  TreatAsAtomicUnit=on
  Tune Variable : TuneVar/TuneVar  TuneName=ForwardDownmixThreshold  SpecifyMaxSize=off  VariableDim=1 (Row)  MaxSize=[1 1]  TunabilityNumber=1  MinValue=[0]  MaxValue=[1]  TriggerInit=[-80 25 90 75]  MaskValue=tuneStruct.ForwardDownmixThreshold
      settings: SourceProductName=Bose Talaria
  wires:
  Tune Variable/1 -> Trivial Translation/1(ForwardDownmixThreshold)  "ForwardDownmixThreshold"
  Trivial Translation/1(TOP) -> TOP/1
  TranslateTrigger/1 -> Trivial Translation/Trigger

== system Model_TranslationEngine64/ModelPreAmp/DecRate/Medusa5H1/MedusaHoligram/Medusa5H1 Part 3/On/VLS Gains Computation/VLS Gains Drv/Fade Tuning/Foward Downmix Max ==
  TOP : TOP/TOP  TriggerInit=[440 20 585 80]  TopName=ForwardDownmixMax  DataTypeOut=single  BankNumber=0  PreOverlay=false  PostOverlay=false  Role=Automatic
      settings: SourceProductName=Bose Talaria
  TranslateTrigger : TuneVar/TranslateTrigger  TriggerInit=[286 -100 324 -45]
      settings: SourceProductName=Bose Talaria
  Trivial Translation : MATLAB Function  TreatAsAtomicUnit=on
  Tune Variable : TuneVar/TuneVar  TuneName=ForwardDownmixMax  SpecifyMaxSize=off  VariableDim=1 (Row)  MaxSize=[1 1]  TunabilityNumber=1  MinValue=[0]  MaxValue=[1]  TriggerInit=[-70 25 100 75]  MaskValue=tuneStruct.ForwardDownmixMax
      settings: SourceProductName=Bose Talaria
  wires:
  Tune Variable/1 -> Trivial Translation/1(ForwardDownmixMax)  "ForwardDownmixMax"
  Trivial Translation/1(TOP) -> TOP/1
  TranslateTrigger/1 -> Trivial Translation/Trigger

== system Model_TranslationEngine64/ModelPreAmp/DecRate/Medusa5H1/MedusaHoligram/Medusa5H1 Part 3/On/VLS Gains Computation/VLS Gains Drv/SLC Tuning/Detent Level ==
  TOP : TOP/TOP  TriggerInit=[405 22 635 78]  TopName=DetentLevel  DataTypeOut=single  BankNumber=0  PreOverlay=false  PostOverlay=false  Role=Automatic
      settings: SourceProductName=Bose Talaria
  TranslateTrigger : TuneVar/TranslateTrigger  TriggerInit=[266 -100 304 -45]
      settings: SourceProductName=Bose Talaria
  Trivial Translation : MATLAB Function  TreatAsAtomicUnit=on
  Tune Variable : TuneVar/TuneVar  TuneName=DetentLevel  SpecifyMaxSize=off  VariableDim=1 (Row)  MaxSize=[1 1]  TunabilityNumber=1  MinValue=[0]  MaxValue=[1]  TriggerInit=[-110 25 105 75]  MaskValue=tuneStruct.detentGain
      settings: SourceProductName=Bose Talaria
  wires:
  Tune Variable/1 -> Trivial Translation/1(detentGain)  "DetentLevel"
  Trivial Translation/1(TOP) -> TOP/1
  TranslateTrigger/1 -> Trivial Translation/Trigger

== system Model_TranslationEngine64/ModelPreAmp/DecRate/Medusa5H1/MedusaHoligram/Medusa5H1 Part 3/On/VLS Gains Computation/VLS Gains Drv/SLC Tuning/Interpolation Method ==
  TOP : TOP/TOP  TriggerInit=[440 20 585 80]  TopName=Interpolation_Method  DataTypeOut=single  BankNumber=0  PreOverlay=false  PostOverlay=false  Role=Automatic
      settings: SourceProductName=Bose Talaria
  TranslateTrigger : TuneVar/TranslateTrigger  TriggerInit=[306 -100 344 -45]
      settings: SourceProductName=Bose Talaria
  Trivial Translation : MATLAB Function  TreatAsAtomicUnit=on
  Tune Variable : TuneVar/TuneVar  TuneName=Interpolation_Method  SpecifyMaxSize=off  VariableDim=1 (Row)  MaxSize=[1 1]  TunabilityNumber=2  MinValue=[0]  MaxValue=[1]  TriggerInit=[-40 25 130 75]  MaskValue=tuneStruct.interpolationMethod
      settings: SourceProductName=Bose Talaria
  wires:
  Tune Variable/1 -> Trivial Translation/1(interpolationMethod)  "Interpolation_Method"
  Trivial Translation/1(TOP) -> TOP/1
  TranslateTrigger/1 -> Trivial Translation/Trigger

== system Model_TranslationEngine64/ModelPreAmp/DecRate/Medusa5H1/MedusaHoligram/Medusa5H1 Part 3/On/VLS Gains Computation/VLS Gains Drv/SLC Tuning/Max Level ==
  TOP : TOP/TOP  TriggerInit=[425 22 630 78]  TopName=MaxLevel  DataTypeOut=single  BankNumber=0  PreOverlay=false  PostOverlay=false  Role=Automatic
      settings: SourceProductName=Bose Talaria
  TranslateTrigger : TuneVar/TranslateTrigger  TriggerInit=[306 -100 344 -45]
      settings: SourceProductName=Bose Talaria
  Trivial Translation : MATLAB Function  TreatAsAtomicUnit=on
  Tune Variable : TuneVar/TuneVar  TuneName=MaxLevel  SpecifyMaxSize=off  VariableDim=1 (Row)  MaxSize=[1 1]  TunabilityNumber=1  MinValue=[0]  MaxValue=[1]  TriggerInit=[-55 25 145 75]  MaskValue=tuneStruct.maxGain
      settings: SourceProductName=Bose Talaria
  wires:
  Tune Variable/1 -> Trivial Translation/1(maxGain)  "MaxLevel"
  Trivial Translation/1(TOP) -> TOP/1
  TranslateTrigger/1 -> Trivial Translation/Trigger

== system Model_TranslationEngine64/ModelPreAmp/DecRate/Medusa5H1/MedusaHoligram/Medusa5H1 Part 3/On/VLS Gains Computation/VLS Gains Drv/SLC Tuning/Min Level ==
  TOP : TOP/TOP  TriggerInit=[360 17 565 73]  TopName=MinLevel  DataTypeOut=single  BankNumber=0  PreOverlay=false  PostOverlay=false  Role=Automatic
      settings: SourceProductName=Bose Talaria
  TranslateTrigger : TuneVar/TranslateTrigger  TriggerInit=[231 -105 269 -50]
      settings: SourceProductName=Bose Talaria
  Trivial Translation : MATLAB Function  TreatAsAtomicUnit=on
  Tune Variable : TuneVar/TuneVar  TuneName=MinLevel  SpecifyMaxSize=off  VariableDim=1 (Row)  MaxSize=[1 1]  TunabilityNumber=1  MinValue=[0]  MaxValue=[1]  TriggerInit=[-120 20 65 70]  MaskValue=tuneStruct.minGain
      settings: SourceProductName=Bose Talaria
  wires:
  Tune Variable/1 -> Trivial Translation/1(minGain)  "MinLevel"
  Trivial Translation/1(TOP) -> TOP/1
  TranslateTrigger/1 -> Trivial Translation/Trigger

== system Model_TranslationEngine64/ModelPreAmp/DecRate/Medusa5H1/MedusaHoligram/Medusa5H1 Part 3/On/VLS Gains Computation/VLS Gains Pax/Fade Tuning/Backward Downmix Max ==
  TOP : TOP/TOP  TriggerInit=[440 20 585 80]  TopName=BackwardDownmixMax  DataTypeOut=single  BankNumber=0  PreOverlay=false  PostOverlay=false  Role=Automatic
      settings: SourceProductName=Bose Talaria
  TranslateTrigger : TuneVar/TranslateTrigger  TriggerInit=[286 -100 324 -45]
      settings: SourceProductName=Bose Talaria
  Trivial Translation : MATLAB Function  TreatAsAtomicUnit=on
  Tune Variable : TuneVar/TuneVar  TuneName=BackwardDownmixMax  SpecifyMaxSize=off  VariableDim=1 (Row)  MaxSize=[1 1]  TunabilityNumber=1  MinValue=[0]  MaxValue=[1]  TriggerInit=[-65 25 105 75]  MaskValue=tuneStruct.BackwardDownmixMax
      settings: SourceProductName=Bose Talaria
  wires:
  Tune Variable/1 -> Trivial Translation/1(BackwardDownmixMax)  "BackwardDownmixMax"
  Trivial Translation/1(TOP) -> TOP/1
  TranslateTrigger/1 -> Trivial Translation/Trigger

== system Model_TranslationEngine64/ModelPreAmp/DecRate/Medusa5H1/MedusaHoligram/Medusa5H1 Part 3/On/VLS Gains Computation/VLS Gains Pax/Fade Tuning/Backward Downmix Threshold ==
  TOP : TOP/TOP  TriggerInit=[440 20 585 80]  TopName=BackwardDownmixThreshold  DataTypeOut=single  BankNumber=0  PreOverlay=false  PostOverlay=false  Role=Automatic
      settings: SourceProductName=Bose Talaria
  TranslateTrigger : TuneVar/TranslateTrigger  TriggerInit=[306 -100 344 -45]
      settings: SourceProductName=Bose Talaria
  Trivial Translation : MATLAB Function  TreatAsAtomicUnit=on
  Tune Variable : TuneVar/TuneVar  TuneName=BackwardDownmixThreshold  SpecifyMaxSize=off  VariableDim=1 (Row)  MaxSize=[1 1]  TunabilityNumber=1  MinValue=[0]  MaxValue=[1]  TriggerInit=[-75 25 95 75]  MaskValue=tuneStruct.BackwardDownmixThreshold
      settings: SourceProductName=Bose Talaria
  wires:
  Tune Variable/1 -> Trivial Translation/1(BackwardDownmixThreshold)  "BackwardDownmixThreshold"
  Trivial Translation/1(TOP) -> TOP/1
  TranslateTrigger/1 -> Trivial Translation/Trigger

== system Model_TranslationEngine64/ModelPreAmp/DecRate/Medusa5H1/MedusaHoligram/Medusa5H1 Part 3/On/VLS Gains Computation/VLS Gains Pax/Fade Tuning/Downmix Weights ==
  TOP : TOP/TOP  TriggerInit=[385 17 610 83]  TopName=DownmixWeights  DataTypeOut=single  BankNumber=0  PreOverlay=false  PostOverlay=false  Role=Automatic
      settings: SourceProductName=Bose Talaria
  TranslateTrigger : TuneVar/TranslateTrigger  TriggerInit=[266 -100 304 -45]
      settings: SourceProductName=Bose Talaria
  Trivial Translation : MATLAB Function  TreatAsAtomicUnit=on
  Tune Variable : TuneVar/TuneVar  TuneName=DownmixWeights  SpecifyMaxSize=off  VariableDim=1 (Row)  MaxSize=[1 1]  TunabilityNumber=1  MinValue=[0]  MaxValue=[1]  TriggerInit=[-80 25 150 75]  MaskValue=tuneStruct.downmix_wts
      settings: SourceProductName=Bose Talaria
  wires:
  Tune Variable/1 -> Trivial Translation/1(downmix_wts)  "DownmixWeights"
  Trivial Translation/1(TOP) -> TOP/1
  TranslateTrigger/1 -> Trivial Translation/Trigger

== system Model_TranslationEngine64/ModelPreAmp/DecRate/Medusa5H1/MedusaHoligram/Medusa5H1 Part 3/On/VLS Gains Computation/VLS Gains Pax/Fade Tuning/Forward Downmix Threshold ==
  TOP : TOP/TOP  TriggerInit=[440 20 585 80]  TopName=ForwardDownmixThreshold  DataTypeOut=single  BankNumber=0  PreOverlay=false  PostOverlay=false  Role=Automatic
      settings: SourceProductName=Bose Talaria
  TranslateTrigger : TuneVar/TranslateTrigger  TriggerInit=[291 -100 329 -45]
      settings: SourceProductName=Bose Talaria
  Trivial Translation : MATLAB Function  TreatAsAtomicUnit=on
  Tune Variable : TuneVar/TuneVar  TuneName=ForwardDownmixThreshold  SpecifyMaxSize=off  VariableDim=1 (Row)  MaxSize=[1 1]  TunabilityNumber=1  MinValue=[0]  MaxValue=[1]  TriggerInit=[-80 25 90 75]  MaskValue=tuneStruct.ForwardDownmixThreshold
      settings: SourceProductName=Bose Talaria
  wires:
  Tune Variable/1 -> Trivial Translation/1(ForwardDownmixThreshold)  "ForwardDownmixThreshold"
  Trivial Translation/1(TOP) -> TOP/1
  TranslateTrigger/1 -> Trivial Translation/Trigger
